simulink model "SWC_FDC_type"  (R2021b)
settings: Solver=FixedStepDiscrete  StartTime=0.0  StopTime=10.0  FixedStep=0.001  RelTol=1e-3
values from neighbouring files (symbols this model uses):
  DID_VCUKey = uint16(0x0202)    [vcu_local_hdr.m]
  DID_XWD = uint16(513)    [vcu_local_hdr.m]
  DIDLen_APSFunConfig = uint16(16)    [vcu_local_hdr.m]
  DIDLen_AutoLock = uint16(1)    [vcu_local_hdr.m]
  DIDLen_DKCKey = uint16(8)    [vcu_local_hdr.m]
  DIDLen_DRLDis = uint16(1)    [vcu_local_hdr.m]
  DIDLen_DynoMode = uint16(1)    [vcu_local_hdr.m]
  DIDLen_FMHTimer = uint16(1)    [vcu_local_hdr.m]
  DIDLen_LFLowPresThre = uint16(1)    [vcu_local_hdr.m]
  DIDLen_LFSensorID = uint16(4)    [vcu_local_hdr.m]
  DIDLen_LRLowPresThre = uint16(1)    [vcu_local_hdr.m]
  DIDLen_LRSensorID = uint16(4)    [vcu_local_hdr.m]
  DIDLen_RFLowPresThre = uint16(1)    [vcu_local_hdr.m]
  DIDLen_RFSensorID = uint16(4)    [vcu_local_hdr.m]
  DIDLen_RRLowPresThre = uint16(1)    [vcu_local_hdr.m]
  DIDLen_RRSensorID = uint16(4)    [vcu_local_hdr.m]
  DIDLen_SensorMode = uint16(1)    [vcu_local_hdr.m]
  DIDLen_TireSize = uint16(16)    [vcu_local_hdr.m]
  DIDLen_TPMSLearnSta = uint16(1)    [vcu_local_hdr.m]
  DIDLen_TurnLampFLThreCurr = uint16(1)    [vcu_local_hdr.m]
  DIDLen_TurnLampFRThreCurr = uint16(1)    [vcu_local_hdr.m]
  DIDLen_TurnLampRLThreCurr = uint16(1)    [vcu_local_hdr.m]
  DIDLen_TurnLampRRThreCurr = uint16(1)    [vcu_local_hdr.m]
  DIDLen_USSConfig = uint16(16)    [vcu_local_hdr.m]
  DIDLen_WhlPres = uint16(4)    [vcu_local_hdr.m]
  DIDLen_WhlSensorBattSta = uint16(1)    [vcu_local_hdr.m]
  DIDLen_WhlTmp = uint16(4)    [vcu_local_hdr.m]
  DIDLen_XWDMode = uint16(1)    [vcu_local_hdr.m]
  DIDNum_APSFunConfig = uint16(0x0903)    [vcu_local_hdr.m]
  DIDNum_AutoLock = uint16(0x0306)    [vcu_local_hdr.m]
  DIDNum_DKCKey = uint16(0x0202)    [vcu_local_hdr.m]
  DIDNum_DRLDis = uint16(0x0307)    [vcu_local_hdr.m]
  DIDNum_DynoMode = uint16(0x0203)    [vcu_local_hdr.m]
  DIDNum_FMHTimer = uint16(0x0305)    [vcu_local_hdr.m]
  DIDNum_LFLowPresThre = uint16(0x0B08)    [vcu_local_hdr.m]
  DIDNum_LFSensorID = uint16(0x0B01)    [vcu_local_hdr.m]
  DIDNum_LRLowPresThre = uint16(0x0B0A)    [vcu_local_hdr.m]
  DIDNum_LRSensorID = uint16(0x0B03)    [vcu_local_hdr.m]
  DIDNum_RFLowPresThre = uint16(0x0B09)    [vcu_local_hdr.m]
  DIDNum_RFSensorID = uint16(0x0B02)    [vcu_local_hdr.m]
  DIDNum_RRLowPresThre = uint16(0x0B0B)    [vcu_local_hdr.m]
  DIDNum_RRSensorID = uint16(0x0B04)    [vcu_local_hdr.m]
  DIDNum_SensorMode = uint16(0x0B0C)    [vcu_local_hdr.m]
  DIDNum_TireSize = uint16(0x0902)    [vcu_local_hdr.m]
  DIDNum_TPMSLearnSta = uint16(0x0B0D)    [vcu_local_hdr.m]
  DIDNum_TurnLampFLThreCurr = uint16(0x0303)    [vcu_local_hdr.m]
  DIDNum_TurnLampFRThreCurr = uint16(0x0301)    [vcu_local_hdr.m]
  DIDNum_TurnLampRLThreCurr = uint16(0x0304)    [vcu_local_hdr.m]
  DIDNum_TurnLampRRThreCurr = uint16(0x0302)    [vcu_local_hdr.m]
  DIDNum_USSConfig = uint16(0x0901)    [vcu_local_hdr.m]
  DIDNum_WhlPres = uint16(0x0B05)    [vcu_local_hdr.m]
  DIDNum_WhlSensorBattSta = uint16(0x0B07)    [vcu_local_hdr.m]
  DIDNum_WhlTmp = uint16(0x0B06)    [vcu_local_hdr.m]
  DIDNum_XWDMode = uint16(0x0201)    [vcu_local_hdr.m]
  DIDVCUKeyLength = uint16(8)    [vcu_local_hdr.m]
  ENUM_DRIVETRAIN_AWD = uint8(  2  )    [vcu_local_hdr.m]
  ENUM_DRIVETRAIN_FWD = uint8(  1  )    [vcu_local_hdr.m]
  ENUM_DRIVETRAIN_RWD = uint8(  0  )    [vcu_local_hdr.m]
  ENUM_TPMSLearnStatus_LEARNED = uint8(  1  )    [vcu_local_hdr.m]
  ENUM_TPMSLearnStatus_LEARNFAIL = uint8(  2  )    [vcu_local_hdr.m]
  ENUM_TPMSLearnStatus_NOTLEARN = uint8(  0  )    [vcu_local_hdr.m]
  ENUM_TPMSSTA_FAT = uint8(  8  )    [vcu_local_hdr.m]
  ENUM_TPMSSTA_LOWBATTERY = uint8(  2  )    [vcu_local_hdr.m]
  FALSE = boolean( 0 )    [vcu_local_hdr.m]
  ONE_INT = uint8(1)    [vcu_local_hdr.m]
  P_boolean = 0.0    [APPTypes.sldd]
  TRUE = boolean( 1 )    [vcu_local_hdr.m]
  ZERO_FLOAT = single(0)    [vcu_local_hdr.m]
  ZERO_INT = uint8(0)    [vcu_local_hdr.m]
undefined symbols (not defined in the file or in its folder): f32_ApsOutVehSpdSig, KHAL_DKCDecryptEnable_flg_ovrdflg, KHAL_DKCDecryptEnable_flg_ovrdval, KHAL_RandomNumberY1_enum, KHAL_RandomNumberY2_enum, KHAL_RandomNumberY_ovrdflg, KHAL_TPMSRESBUTT_flg_ovrdflg, KHAL_TPMSRESBUTT_flg_ovrdval, R_DIDWriteCDD_CSOP_DIDSet_APSFunConfig, R_DIDWriteCDD_CSOP_DIDSet_AutoLock, R_DIDWriteCDD_CSOP_DIDSet_DKCKey, R_DIDWriteCDD_CSOP_DIDSet_DRLDis, R_DIDWriteCDD_CSOP_DIDSet_DynoMode, R_DIDWriteCDD_CSOP_DIDSet_FMHTimer, R_DIDWriteCDD_CSOP_DIDSet_LFLowPresThre, R_DIDWriteCDD_CSOP_DIDSet_LFSensorID, R_DIDWriteCDD_CSOP_DIDSet_LRLowPresThre, R_DIDWriteCDD_CSOP_DIDSet_LRSensorID, R_DIDWriteCDD_CSOP_DIDSet_RFLowPresThre, R_DIDWriteCDD_CSOP_DIDSet_RFSensorID, R_DIDWriteCDD_CSOP_DIDSet_RRLowPresThre, R_DIDWriteCDD_CSOP_DIDSet_RRSensorID, R_DIDWriteCDD_CSOP_DIDSet_SensorMode, R_DIDWriteCDD_CSOP_DIDSet_TireSize, R_DIDWriteCDD_CSOP_DIDSet_TPMSLearnSta, R_DIDWriteCDD_CSOP_DIDSet_TurnLampFLThreCurr, R_DIDWriteCDD_CSOP_DIDSet_TurnLampFRThreCurr, R_DIDWriteCDD_CSOP_DIDSet_TurnLampRLThreCurr, R_DIDWriteCDD_CSOP_DIDSet_TurnLampRRThreCurr, R_DIDWriteCDD_CSOP_DIDSet_USSConfig, R_DIDWriteCDD_CSOP_DIDSet_WhlPres, R_DIDWriteCDD_CSOP_DIDSet_WhlSensorBattSta, R_DIDWriteCDD_CSOP_DIDSet_WhlTmp, R_DIDWriteCDD_CSOP_DIDSet_XWDMode, R_E2E_CAN3_VCU1_CSOP_Write_CAN3_VCU1, R_E2E_CAN3_VCU1_toNIDEC_CSOP_Write_CAN3_VCU1_toNIDEC, R_E2E_CAN4_VCU1_CSOP_Write_CAN4_VCU1, R_FDCCDD_Inner_CSOP_FDC_AppCallSleep, R_HALINCDD_CSOP_PAS_Handler, R_HALINCDD_CSOP_UDS_Main, R_HALOUT_APS_CSOP_ApsOutput, R_HALOUTCDD_CSOP_AppNmStateReq, R_HALOUTCDD_CSOP_SetAcoreRebootCmdACK, R_HALOUTCDD_CSOP_SetSysPwrStat, R_HALOUTCDD_CSOP_SleepRequest, R_IOExpOUT_CDD_CSOP_IOExpSetVal, R_J1939_CAN1_CFGEM1_BAM_CSOP_Write_CAN1_CFGEM1_BAM, R_J1939_CAN1_CFGEM1_DT_CSOP_Write_CAN1_CFGEM1_DT, R_NVMReadCDD_Inner_NVM_ReadOperation, R_NVMWriteCDD_Inner_NVM_WriteOperation, R_UDSCDD_CSOP_DdmRestartOperationCycle, R_WDGCDD_CSOP_Call_Watchdog, R_WDGCDD_CSOP_Call_WDG_AppEnd, R_WDGCDD_CSOP_Call_WDG_AppStart, u16_DIDLen_APSFunConfig, u16_DIDLen_AutoLock, u16_DIDLen_DKCKey, u16_DIDLen_DRLDis, u16_DIDLen_DynoMode, u16_DIDLen_FMHTimer ... (+83)
libraries: simulink x215, FVT_lib x143, hcu_lib x19, hdlsllib x9, app x1, halin x1, halout x1, inp x1, outp x1
(part 11 of 13)

== system SWC_FDC_type/run_SWC_FDC_RxTx_5ms_sys/Halin_CDD/Halin_SYS/Flashfdefog_Verify ==
  In1 : Inport
  Compare To Constant : simulink/Logic and Bit Operations/Compare To Constant  relop=>  const=1  OutDataTypeStr=boolean
  Compare To Constant1 : simulink/Logic and Bit Operations/Compare To Constant  relop=<  const=0  OutDataTypeStr=boolean
  Constant : Constant  Value=ZERO_INT
  Logical Operator : Logic  Operator=OR  AllPortsSameDT=off  OutDataTypeStr=boolean
  Switch : Switch  Criteria=u2 > Threshold
  Out1 : Outport
  wires:
  In1/1 -> Switch/3, Compare To Constant1/1, Compare To Constant/1
  Constant/1 -> Switch/1
  Switch/1 -> Out1/1
  Logical Operator/1 -> Switch/2
  Compare To Constant/1 -> Logical Operator/1
  Compare To Constant1/1 -> Logical Operator/2

== system SWC_FDC_type/run_SWC_FDC_RxTx_5ms_sys/Halin_CDD/Halin_SYS/FlashsigRecircSt_Verify ==
  In1 : Inport
  Compare To Constant : simulink/Logic and Bit Operations/Compare To Constant  relop=>  const=1  OutDataTypeStr=boolean
  Compare To Constant1 : simulink/Logic and Bit Operations/Compare To Constant  relop=<  const=0  OutDataTypeStr=boolean
  Constant : Constant  Value=ZERO_INT
  Logical Operator : Logic  Operator=OR  AllPortsSameDT=off  OutDataTypeStr=boolean
  Switch : Switch  Criteria=u2 > Threshold
  Out1 : Outport
  wires:
  Compare To Constant1/1 -> Logical Operator/2
  Compare To Constant/1 -> Logical Operator/1
  Logical Operator/1 -> Switch/2
  Switch/1 -> Out1/1
  Constant/1 -> Switch/1
  In1/1 -> Compare To Constant/1, Compare To Constant1/1, Switch/3

== system SWC_FDC_type/run_SWC_FDC_RxTx_5ms_sys/Halin_CDD/Halin_SYS/FlashsigSetTempZon1St_Verify ==
  In1 : Inport
  Compare To Constant : simulink/Logic and Bit Operations/Compare To Constant  relop=>  const=32  OutDataTypeStr=boolean
  Compare To Constant1 : simulink/Logic and Bit Operations/Compare To Constant  relop=<  const=17  OutDataTypeStr=boolean
  Constant : Constant  Value=25
  Logical Operator : Logic  Operator=OR  AllPortsSameDT=off  OutDataTypeStr=boolean
  Switch : Switch  Criteria=u2 > Threshold
  Out1 : Outport
  wires:
  In1/1 -> Switch/3, Compare To Constant1/1, Compare To Constant/1
  Constant/1 -> Switch/1
  Switch/1 -> Out1/1
  Logical Operator/1 -> Switch/2
  Compare To Constant/1 -> Logical Operator/1
  Compare To Constant1/1 -> Logical Operator/2

== system SWC_FDC_type/run_SWC_FDC_RxTx_5ms_sys/Halin_CDD/Halin_SYS/FlashsigSetTempZon2StM_Verify ==
  In1 : Inport
  Compare To Constant : simulink/Logic and Bit Operations/Compare To Constant  relop=>  const=32  OutDataTypeStr=boolean
  Compare To Constant1 : simulink/Logic and Bit Operations/Compare To Constant  relop=<  const=17  OutDataTypeStr=boolean
  Constant : Constant  Value=25
  Logical Operator : Logic  Operator=OR  AllPortsSameDT=off  OutDataTypeStr=boolean
  Switch : Switch  Criteria=u2 > Threshold
  Out1 : Outport
  wires:
  Compare To Constant1/1 -> Logical Operator/2
  Compare To Constant/1 -> Logical Operator/1
  Logical Operator/1 -> Switch/2
  Switch/1 -> Out1/1
  Constant/1 -> Switch/1
  In1/1 -> Compare To Constant/1, Compare To Constant1/1, Switch/3

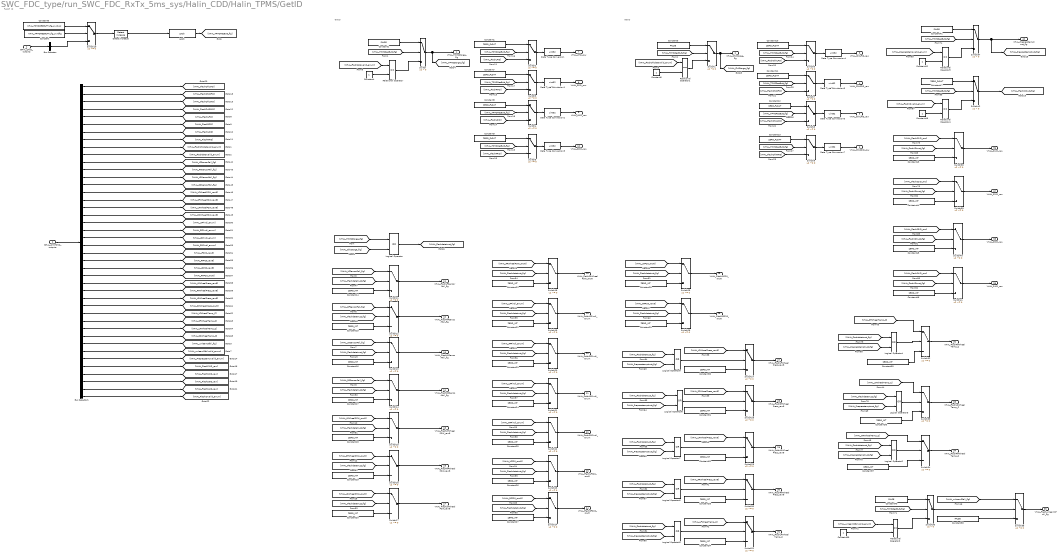
== system SWC_FDC_type/run_SWC_FDC_RxTx_5ms_sys/Halin_CDD/Halin_TPMS/GetID ==
  note: FLASH ID
  note: GetID
  note: GetID
  BHAL_CAN2_outputs : Inport
  BHAL_SYSTPMS_outputs : Inport  Port=2
  Bus Selector : BusSelector  OutputSignals=VHAL_TPMSResButt_flg
  Bus Selector1 : BusSelector  OutputSignals=VHAL_FlashChkLFID_raw,VHAL_FlashChkRFID_raw,VHAL_FlashChkLRID_raw,VHAL_FlashChkRRID_raw,VHAL_FlashLFID_raw,VHAL_FlashRFID_raw,VHAL_FlashLRID_raw,VHAL_FlashRRID_raw,VHAL_Flashchkdatavalid_enum,VHAL_Flashdatavalid_enum,VHAL_LFSensorFail_flg,VHAL_RFSensorFail_flg,VHAL_LRSensorFail_flg,VHAL_RRSensorFail_flg,VHAL_LFWheelPSW_raw8,VHAL_RFWheelPSW_raw8,VHAL_LRWheelPSW_raw8,VHAL_RRWheelPSW_raw8,VHAL_LFPindi_enum,VHAL_RFPindi_enum,VHAL_LRPindi_enum,VHAL_RRPindi_enum,VHAL_LFP20_raw8,VHAL_RFP20_raw8,VHAL_LRP20_raw8,VHAL_RRP20_raw8,VHAL_LFWheelPress_raw8,VHAL_RFWheelPress_raw8,VHAL_LRWheelPress_raw8,VHAL_RRWheelPress_raw8,VHAL_LFWheelTemp_C,VHAL_RFWheelTemp_C,VHAL_LRWheelTemp_C,VHAL_RRWheelTemp_C,VHAL_unlearnSfali_flg,VHAL_unlearnSfailvalid_enum,VHAL_Prepresstempvalid_enum,VHAL_FlashS1ID_raw,VHAL_FlashS2ID_raw,VHAL_FlashS3ID_raw,VHAL_FlashS4ID_raw,VHAL_FlashIDvalid_enum
  Constant : Constant  Value=KHAL_TPMSRESBUTT_flg_ovrdflg
  Constant{1,7..13,47} (9 alike) : Constant  Value=ZERO_FLOAT
  Constant{14..37,43..46} (28 alike) : Constant  Value=ZERO_INT
  Constant{2..3,38,40..41} (5 alike) : Constant  Value=FALSE
  Constant{4..5,39,42,48} (5 alike) : Constant
  Constant6 : Constant  Value=KHAL_TPMSRESBUTT_flg_ovrdval
  Data Type Conversion{,1..7} (8 alike) : DataTypeConversion  OutDataTypeStr=uint32
  Detect Increase : simulink/Logic and Bit Operations/Detect Increase  vinit=0.0  OutDataTypeStr=boolean
  Latch : hcu_lib/Basic_Blocks/Latch
  Logical Operator{,2..9} (9 alike) : Logic  Operator=OR  AllPortsSameDT=off  OutDataTypeStr=boolean
  Relational Operator{,1..4} (5 alike) : RelationalOperator  Operator===  OutDataTypeStr=boolean  RndMeth=Simplest
  Switch{,36..37,42} (4 alike) : Switch  Criteria=u2 > Threshold
  Switch{1..35,38..41} (39 alike) : Switch  Criteria=u2 ~= 0
  VHAL_TPMSStorge_flg : Outport
  VHAL_ChkStorge_flg : Outport  Port=2
  VHAL_ChkLFID_raw : Outport  Port=3
  VHAL_ChkRFID_raw : Outport  Port=4
  VHAL_ChkLRID_raw : Outport  Port=5
  VHAL_ChkRRID_raw : Outport  Port=6
  VHAL_LFID_raw : Outport  Port=7
  VHAL_RFID_raw : Outport  Port=8
  VHAL_LRID_raw : Outport  Port=9
  VHAL_RRID_raw : Outport  Port=10
  VHAL_FlashLFSensorFail_flg : Outport  Port=11
  VHAL_FlashRFSensorFail_flg : Outport  Port=12
  VHAL_FlashLRSensorFail_flg : Outport  Port=13
  VHAL_FlashRRSensorFail_flg : Outport  Port=14
  VHAL_FlashLFWheelPSW_raw8 : Outport  Port=15
  VHAL_FlashRFWheelPSW_raw8 : Outport  Port=16
  VHAL_FlashLRWheelPSW_raw8 : Outport  Port=17
  VHAL_FlashRRWheelPSW_raw8 : Outport  Port=18
  VHAL_FlashLFPindi_enum : Outport  Port=19
  VHAL_FlashRFPindi_enum : Outport  Port=20
  VHAL_FlashLRPindi_enum : Outport  Port=21
  VHAL_FlashRRPindi_enum : Outport  Port=22
  VHAL_FlashLFP20_raw8 : Outport  Port=23
  VHAL_FlashRFP20_raw8 : Outport  Port=24
  VHAL_FlashLRP20_raw8 : Outport  Port=25
  VHAL_FlashRRP20_raw8 : Outport  Port=26
  VHAL_FlashLFWheelPress_raw8 : Outport  Port=27
  VHAL_FlashRFWheelPress_raw8 : Outport  Port=28
  VHAL_FlashLRWheelPress_raw8 : Outport  Port=29
  VHAL_FlashRRWheelPress_raw8 : Outport  Port=30
  VHAL_FlashLFWheelTemp_C : Outport  Port=31
  VHAL_FlashRFWheelTemp_C : Outport  Port=32
  VHAL_FlashLRWheelTemp_C : Outport  Port=33
  VHAL_FlashRRWheelTemp_C : Outport  Port=34
  VHAL_FlashunlearnSfali_flg : Outport  Port=35
  VHAL_S1ID_raw : Outport  Port=36
  VHAL_S2ID_raw : Outport  Port=37
  VHAL_S3ID_raw : Outport  Port=38
  VHAL_S4ID_raw : Outport  Port=39
  VHAL_Prepresstemptrust_flg : Outport  Port=40
  wires:
  BHAL_CAN2_outputs/1 -> Bus Selector/1
  Latch/1 -> [VHAL_TPMSResButt_flg]
  [VHAL_TPMSResButt_flg] -> Switch4/2
  [VHAL_TPMSResButt_flg] -> Switch3/2
  [VHAL_FlashChkLFID] -> Switch6/3
  Switch3/1 -> Data Type Conversion1/1
  [VHAL_FlashRFID] -> Switch3/3
  Constant12/1 -> Switch8/1
  Constant9/1 -> Switch5/1
  [VHAL_FlashRRID] -> Switch5/3
  Constant1/1 -> Switch2/1
  Constant7/1 -> Switch3/1
  [VHAL_TPMSResButt_flg] -> Switch9/2
  [VHAL_TPMSResButt_flg] -> Switch2/2
  [VHAL_FlashLRID] -> Switch4/3
  Constant8/1 -> Switch4/1
  Switch2/1 -> Data Type Conversion/1
  [VHAL_TPMSResButt_flg] -> Switch5/2
  Switch4/1 -> Data Type Conversion2/1
  [VHAL_FlashChkLRID] -> Switch8/3
  [VHAL_FlashChkRRID] -> Switch9/3
  Constant10/1 -> Switch6/1
  Constant11/1 -> Switch7/1
  Switch8/1 -> Data Type Conversion6/1
  [VHAL_TPMSResButt_flg] -> Switch6/2
  Switch6/1 -> Data Type Conversion4/1
  Switch9/1 -> Data Type Conversion7/1
  Constant13/1 -> Switch9/1
  Switch7/1 -> Data Type Conversion5/1
  [VHAL_TPMSResButt_flg] -> Switch8/2
  [VHAL_TPMSResButt_flg] -> Switch7/2
  Switch5/1 -> Data Type Conversion3/1
  [VHAL_FlashChkRFID] -> Switch7/3
  [VHAL_FlashLFID] -> Switch2/3
  Switch10/1 -> Detect Increase/1
  Constant/1 -> Switch10/2
  Constant6/1 -> Switch10/1
  Bus Selector/1 -> Switch10/3  "<VHAL_TPMSResButt_flg>"
  [VHAL_TPMSResButt_flg] -> Switch/2
  Switch/1 -> [VHAL_TPMSStorge_flg], VHAL_TPMSStorge_flg/1
  Constant2/1 -> Switch/1
  Constant3/1 -> Switch1/1
  Switch1/1 -> [VHAL_ChkStorge_flg], VHAL_ChkStorge_flg/1
  [VHAL_TPMSResButt_flg] -> Switch1/2
  [VHAL_Flashdatavalid_enum] -> Relational Operator/1
  Relational Operator/1 -> Switch/3
  Constant4/1 -> Relational Operator/2
  Constant5/1 -> Relational Operator1/2
  Relational Operator1/1 -> Switch1/3
  [VHAL_Flashchkdatavalid_enum] -> Relational Operator1/1
  [VHAL_TPMSStorge_flg] -> Logical Operator/1
  [VHAL_ChkStorge_flg] -> Logical Operator/2
  Logical Operator/1 -> [VHAL_Flashdatatrust_flg]
  [VHAL_Flashdatatrust_flg] -> Switch11/2
  [VHAL_LFSensorFail_flg] -> Switch11/1
  Constant14/1 -> Switch11/3
  Switch11/1 -> VHAL_FlashLFSensorFail_flg/1
  Constant15/1 -> Switch12/3
  [VHAL_Flashdatatrust_flg] -> Switch12/2
  Constant16/1 -> Switch13/3
  [VHAL_Flashdatatrust_flg] -> Switch13/2
  Constant17/1 -> Switch14/3
  [VHAL_Flashdatatrust_flg] -> Switch14/2
  Constant18/1 -> Switch15/3
  [VHAL_Flashdatatrust_flg] -> Switch15/2
  Constant19/1 -> Switch16/3
  [VHAL_Flashdatatrust_flg] -> Switch16/2
  Constant20/1 -> Switch17/3
  [VHAL_Flashdatatrust_flg] -> Switch17/2
  Constant21/1 -> Switch18/3
  [VHAL_Flashdatatrust_flg] -> Switch18/2
  [VHAL_RFSensorFail_flg] -> Switch12/1
  [VHAL_LRSensorFail_flg] -> Switch13/1
  [VHAL_RRSensorFail_flg] -> Switch14/1
  [VHAL_LFWheelPSW_raw8] -> Switch15/1
  [VHAL_RFWheelPSW_raw8] -> Switch16/1
  [VHAL_LRWheelPSW_raw8] -> Switch17/1
  [VHAL_RRWheelPSW_raw8] -> Switch18/1
  Constant22/1 -> Switch19/3
  [VHAL_Flashdatatrust_flg] -> Switch19/2
  Constant23/1 -> Switch20/3
  [VHAL_Flashdatatrust_flg] -> Switch20/2
  Constant24/1 -> Switch21/3
  [VHAL_Flashdatatrust_flg] -> Switch21/2
  Constant25/1 -> Switch22/3
  [VHAL_Flashdatatrust_flg] -> Switch22/2
  [VHAL_LFPindi_enum] -> Switch19/1
  [VHAL_RFPindi_enum] -> Switch20/1
  [VHAL_LRPindi_enum] -> Switch21/1
  [VHAL_RRPindi_enum] -> Switch22/1
  Constant26/1 -> Switch23/3
  [VHAL_Flashdatatrust_flg] -> Switch23/2
  [VHAL_LFP20_raw8] -> Switch23/1
  Constant27/1 -> Switch24/3
  [VHAL_Flashdatatrust_flg] -> Switch24/2
  [VHAL_RFP20_raw8] -> Switch24/1
  Constant28/1 -> Switch25/3
  [VHAL_Flashdatatrust_flg] -> Switch25/2
  [VHAL_LRP20_raw8] -> Switch25/1
  Constant29/1 -> Switch26/3
  [VHAL_Flashdatatrust_flg] -> Switch26/2
  [VHAL_RRP20_raw8] -> Switch26/1
  Constant30/1 -> Switch27/3
  [VHAL_LFWheelPress_raw8] -> Switch27/1
  Constant31/1 -> Switch28/3
  [VHAL_RFWheelPress_raw8] -> Switch28/1
  Constant32/1 -> Switch29/3
  [VHAL_LRWheelPress_raw8] -> Switch29/1
  Constant33/1 -> Switch30/3
  [VHAL_RRWheelPress_raw8] -> Switch30/1
  Constant34/1 -> Switch31/3
  [VHAL_LFWheelTemp_C] -> Switch31/1
  Constant35/1 -> Switch32/3
  [VHAL_RFWheelTemp_C] -> Switch32/1
  Constant36/1 -> Switch33/3
  [VHAL_LRWheelTemp_C] -> Switch33/1
  Constant37/1 -> Switch34/3
  Logical Operator2/1 -> Switch34/2
  Constant38/1 -> Switch35/3
  [VHAL_unlearnSfali_flg] -> Switch35/1
  [VHAL_RRWheelTemp_C] -> Switch34/1
  Switch12/1 -> VHAL_FlashRFSensorFail_flg/1
  Switch13/1 -> VHAL_FlashLRSensorFail_flg/1
  Switch14/1 -> VHAL_FlashRRSensorFail_flg/1
  Switch15/1 -> VHAL_FlashLFWheelPSW_raw8/1
  Switch16/1 -> VHAL_FlashRFWheelPSW_raw8/1
  Switch17/1 -> VHAL_FlashLRWheelPSW_raw8/1
  Switch18/1 -> VHAL_FlashRRWheelPSW_raw8/1
  Switch19/1 -> VHAL_FlashLFPindi_enum/1
  Switch20/1 -> VHAL_FlashRFPindi_enum/1
  Switch21/1 -> VHAL_FlashLRPindi_enum/1
  Switch22/1 -> VHAL_FlashRRPindi_enum/1
  Switch23/1 -> VHAL_FlashLFP20_raw8/1
  Switch24/1 -> VHAL_FlashRFP20_raw8/1
  Switch25/1 -> VHAL_FlashLRP20_raw8/1
  Switch26/1 -> VHAL_FlashRRP20_raw8/1
  Switch27/1 -> VHAL_FlashLFWheelPress_raw8/1
  Switch28/1 -> VHAL_FlashRFWheelPress_raw8/1
  Switch29/1 -> VHAL_FlashLRWheelPress_raw8/1
  Switch30/1 -> VHAL_FlashRRWheelPress_raw8/1
  Switch31/1 -> VHAL_FlashLFWheelTemp_C/1
  Switch32/1 -> VHAL_FlashRFWheelTemp_C/1
  Switch33/1 -> VHAL_FlashLRWheelTemp_C/1
  Switch34/1 -> VHAL_FlashRRWheelTemp_C/1
  [VHAL_unlearnSfailvalid_enum] -> Relational Operator2/1
  Constant39/1 -> Relational Operator2/2
  Constant40/1 -> Switch36/1
  [VHAL_TPMSResButt_flg] -> Switch36/2
  Switch35/1 -> VHAL_FlashunlearnSfali_flg/1
  Switch36/1 -> Switch35/2
  Relational Operator2/1 -> Switch36/3
  Constant42/1 -> Relational Operator3/2
  [VHAL_TPMSResButt_flg] -> Switch37/2
  Constant41/1 -> Switch37/1
  Relational Operator3/1 -> Switch37/3
  [VHAL_Prepresstempvalid_enum] -> Relational Operator3/1
  Switch37/1 -> VHAL_Prepresstemptrust_flg/1, [VHAL_Prepresstemptrust_flg]
  [VHAL_Flashdatatrust_flg] -> Logical Operator2/1
  [VHAL_Prepresstemptrust_flg] -> Logical Operator2/2
  [VHAL_Flashdatatrust_flg] -> Logical Operator3/1
  [VHAL_Prepresstemptrust_flg] -> Logical Operator3/2
  Logical Operator3/1 -> Switch33/2
  [VHAL_Flashdatatrust_flg] -> Logical Operator4/1
  [VHAL_Prepresstemptrust_flg] -> Logical Operator4/2
  Logical Operator4/1 -> Switch32/2
  [VHAL_Flashdatatrust_flg] -> Logical Operator5/1
  [VHAL_Prepresstemptrust_flg] -> Logical Operator5/2
  Logical Operator5/1 -> Switch31/2
  [VHAL_Flashdatatrust_flg] -> Logical Operator6/1
  [VHAL_Prepresstemptrust_flg] -> Logical Operator6/2
  Logical Operator6/1 -> Switch30/2
  [VHAL_Flashdatatrust_flg] -> Logical Operator7/1
  [VHAL_Prepresstemptrust_flg] -> Logical Operator7/2
  Logical Operator7/1 -> Switch29/2
  [VHAL_Flashdatatrust_flg] -> Logical Operator8/1
  [VHAL_Prepresstemptrust_flg] -> Logical Operator8/2
  Logical Operator8/1 -> Switch28/2
  [VHAL_Flashdatatrust_flg] -> Logical Operator9/1
  [VHAL_Prepresstemptrust_flg] -> Logical Operator9/2
  Logical Operator9/1 -> Switch27/2
  Detect Increase/1 -> Latch/1
  Data Type Conversion/1 -> VHAL_LFID_raw/1
  Data Type Conversion1/1 -> VHAL_RFID_raw/1
  Data Type Conversion2/1 -> VHAL_LRID_raw/1
  Data Type Conversion3/1 -> VHAL_RRID_raw/1
  Data Type Conversion4/1 -> VHAL_ChkLFID_raw/1
  Data Type Conversion5/1 -> VHAL_ChkRFID_raw/1
  Data Type Conversion6/1 -> VHAL_ChkLRID_raw/1
  Data Type Conversion7/1 -> VHAL_ChkRRID_raw/1
  Switch42/1 -> [VHAL_FlashIDtrust_flg]
  Constant45/1 -> Switch40/3
  Constant46/1 -> Switch41/3
  Constant44/1 -> Switch39/3
  Switch39/1 -> VHAL_S2ID_raw/1
  [VHAL_FlashS3ID_raw] -> Switch40/1
  [VHAL_FlashS2ID_raw] -> Switch39/1
  [VHAL_FlashS4ID_raw] -> Switch41/1
  Constant43/1 -> Switch38/3
  [VHAL_FlashS1ID_raw] -> Switch38/1
  [VHAL_TPMSResButt_flg] -> Switch42/2
  [VHAL_FlashIDtrust_flg] -> Switch38/2
  Switch41/1 -> VHAL_S4ID_raw/1
  [VHAL_FlashIDtrust_flg] -> Switch39/2
  Constant47/1 -> Switch42/1
  Switch40/1 -> VHAL_S3ID_raw/1
  Constant48/1 -> Relational Operator4/2
  [VHAL_FlashIDtrust_flg] -> Switch41/2
  Switch38/1 -> VHAL_S1ID_raw/1
  [VHAL_FlashIDvalid_enum] -> Relational Operator4/1
  Relational Operator4/1 -> Switch42/3
  [VHAL_FlashIDtrust_flg] -> Switch40/2
  Bus Selector1/35 -> [VHAL_unlearnSfali_flg]  "<VHAL_unlearnSfali_flg>"
  Bus Selector1/4 -> [VHAL_FlashChkRRID]  "<VHAL_FlashChkRRID_raw>"
  Bus Selector1/27 -> [VHAL_LFWheelPress_raw8]  "<VHAL_LFWheelPress_raw8>"
  Bus Selector1/19 -> [VHAL_LFPindi_enum]  "<VHAL_LFPindi_enum>"
  Bus Selector1/21 -> [VHAL_LRPindi_enum]  "<VHAL_LRPindi_enum>"
  Bus Selector1/25 -> [VHAL_LRP20_raw8]  "<VHAL_LRP20_raw8>"
  Bus Selector1/33 -> [VHAL_LRWheelTemp_C]  "<VHAL_LRWheelTemp_C>"
  Bus Selector1/26 -> [VHAL_RRP20_raw8]  "<VHAL_RRP20_raw8>"
  Bus Selector1/18 -> [VHAL_RRWheelPSW_raw8]  "<VHAL_RRWheelPSW_raw8>"
  Bus Selector1/32 -> [VHAL_RFWheelTemp_C]  "<VHAL_RFWheelTemp_C>"
  Bus Selector1/29 -> [VHAL_LRWheelPress_raw8]  "<VHAL_LRWheelPress_raw8>"
  Bus Selector1/8 -> [VHAL_FlashRRID]  "<VHAL_FlashRRID_raw>"
  Bus Selector1/12 -> [VHAL_RFSensorFail_flg]  "<VHAL_RFSensorFail_flg>"
  Bus Selector1/20 -> [VHAL_RFPindi_enum]  "<VHAL_RFPindi_enum>"
  Bus Selector1/11 -> [VHAL_LFSensorFail_flg]  "<VHAL_LFSensorFail_flg>"
  Bus Selector1/24 -> [VHAL_RFP20_raw8]  "<VHAL_RFP20_raw8>"
  Bus Selector1/22 -> [VHAL_RRPindi_enum]  "<VHAL_RRPindi_enum>"
  Bus Selector1/6 -> [VHAL_FlashRFID]  "<VHAL_FlashRFID_raw>"
  Bus Selector1/3 -> [VHAL_FlashChkLRID]  "<VHAL_FlashChkLRID_raw>"
  Bus Selector1/2 -> [VHAL_FlashChkRFID]  "<VHAL_FlashChkRFID_raw>"
  Bus Selector1/37 -> [VHAL_Prepresstempvalid_enum]  "<VHAL_Prepresstempvalid_enum>"
  Bus Selector1/34 -> [VHAL_RRWheelTemp_C]  "<VHAL_RRWheelTemp_C>"
  Bus Selector1/16 -> [VHAL_RFWheelPSW_raw8]  "<VHAL_RFWheelPSW_raw8>"
  Bus Selector1/30 -> [VHAL_RRWheelPress_raw8]  "<VHAL_RRWheelPress_raw8>"
  Bus Selector1/28 -> [VHAL_RFWheelPress_raw8]  "<VHAL_RFWheelPress_raw8>"
  Bus Selector1/14 -> [VHAL_RRSensorFail_flg]  "<VHAL_RRSensorFail_flg>"
  Bus Selector1/38 -> [VHAL_FlashS1ID_raw]  "<VHAL_FlashS1ID_raw>"
  Bus Selector1/41 -> [VHAL_FlashS4ID_raw]  "<VHAL_FlashS4ID_raw>"
  Bus Selector1/10 -> [VHAL_Flashdatavalid_enum]  "<VHAL_Flashdatavalid_enum>"
  Bus Selector1/15 -> [VHAL_LFWheelPSW_raw8]  "<VHAL_LFWheelPSW_raw8>"
  Bus Selector1/5 -> [VHAL_FlashLFID]  "<VHAL_FlashLFID_raw>"
  Bus Selector1/39 -> [VHAL_FlashS2ID_raw]  "<VHAL_FlashS2ID_raw>"
  BHAL_SYSTPMS_outputs/1 -> Bus Selector1/1
  Bus Selector1/9 -> [VHAL_Flashchkdatavalid_enum]  "<VHAL_Flashchkdatavalid_enum>"
  Bus Selector1/1 -> [VHAL_FlashChkLFID]  "<VHAL_FlashChkLFID_raw>"
  Bus Selector1/7 -> [VHAL_FlashLRID]  "<VHAL_FlashLRID_raw>"
  Bus Selector1/36 -> [VHAL_unlearnSfailvalid_enum]  "<VHAL_unlearnSfailvalid_enum>"
  Bus Selector1/23 -> [VHAL_LFP20_raw8]  "<VHAL_LFP20_raw8>"
  Bus Selector1/40 -> [VHAL_FlashS3ID_raw]  "<VHAL_FlashS3ID_raw>"
  Bus Selector1/13 -> [VHAL_LRSensorFail_flg]  "<VHAL_LRSensorFail_flg>"
  Bus Selector1/42 -> [VHAL_FlashIDvalid_enum]  "<VHAL_FlashIDvalid_enum>"
  Bus Selector1/31 -> [VHAL_LFWheelTemp_C]  "<VHAL_LFWheelTemp_C>"
  Bus Selector1/17 -> [VHAL_LRWheelPSW_raw8]  "<VHAL_LRWheelPSW_raw8>"

== system SWC_FDC_type/run_SWC_FDC_RxTx_5ms_sys/Halin_CDD/Halin_TPMS/Subsystem ==
  note: Custom State Judgement
  note: Data Output
  note: Data Valid Judge
  TPMS_DataIn_flg : Inport
  TPMS_RawData : Inport  Port=2
  Add : Sum  Inputs=++++
  Bit Shift : hdlsllib/Logic and Bit Operations/Bit Shift  mode=Shift Left Logical  N=24
  Bit Shift1 : hdlsllib/Logic and Bit Operations/Bit Shift  mode=Shift Left Logical  N=16
  Bit Shift3 : hdlsllib/Logic and Bit Operations/Bit Shift  mode=Shift Left Logical  N=8
  Bitwise NOT : simulink/Logic and Bit Operations/Bitwise Operator  logicop=NOT  UseBitMask=off  BitMask=bin2dec('11011001')  BitMaskRealWorld=Stored Integer
  CRC8_Caculation : Subsystem
  Constant2 : Constant  Value=ENUM_TPMSSTA_LOWBATTERY
  Constant3 : Constant  Value=ENUM_TPMSSTA_FAT
  Constant4 : Constant  Value=TRUE
  Constant5 : Constant  Value=FALSE
  Constant6 : Constant  Value=FALSE
  Constant7 : Constant  Value=TRUE
  Constant8 : Constant  Value=FALSE
  Constant9 : Constant  Value=TRUE
  Data Type Conversion : DataTypeConversion  OutDataTypeStr=uint32
  Data Type Conversion1 : DataTypeConversion  OutDataTypeStr=uint8
  Data Type Conversion2 : DataTypeConversion  OutDataTypeStr=uint8
  Data Type Conversion3 : DataTypeConversion  OutDataTypeStr=uint32
  Data Type Conversion4 : DataTypeConversion  OutDataTypeStr=uint32
  Demux : Demux  Outputs=9
  Demux1 : Demux  Outputs=10
  Equal{,1..3} (4 alike) : RelationalOperator  Operator===  OutDataTypeStr=boolean  RndMeth=Simplest
  Logical Operator : Logic  Inputs=3  AllPortsSameDT=off  OutDataTypeStr=boolean
  Mux : Mux  Inputs=10
  Mux1 : Mux  Inputs=8
  Switch{,1..3} (4 alike) : Switch  Criteria=u2 ~= 0
  Unit Delay : UnitDelay  SampleTime=-1  HasFrameUpgradeWarning=on
  VHAL_TPMSDataIn_flg : Outport
  VHAL_TPMSID_raw : Outport  Port=2
  VHAL_TPMSPressure_raw : Outport  Port=3
  VHAL_TPMSTemp_raw : Outport  Port=4
  VHAL_TPMSSta_enum : Outport  Port=5
  VHAL_TPMSPressureMi_raw : Outport  Port=6
  VHAL_TPMSCRC_crc : Outport  Port=7
  VHAL_TPMSCRCCalc_crc : Outport  Port=8
  VHAL_TPMSFAT_flg : Outport  Port=9
  VHAL_TPMSBattLow_flg : Outport  Port=10
  wires:
  TPMS_DataIn_flg/1 -> Data Type Conversion2/1
  [TPMSData] -> Demux/1
  Bit Shift/1 -> Add/1
  Bit Shift1/1 -> Add/2
  Bit Shift3/1 -> Add/3
  Add/1 -> VHAL_TPMSID_raw/1
  Demux/5 -> [Pressure]  "Pressure"
  Demux/7 -> [Status]  "Sta"
  Demux/8 -> [PressureMirror]  "PressureMirror"
  Demux/9 -> [CRC]  "CRC"
  Demux/1 -> [ID4]  "ID4"
  Demux/2 -> [ID3]  "ID3"
  Demux/3 -> [ID2]  "ID2"
  Demux/4 -> [ID1]  "ID1"
  Demux/6 -> [Temp]  "Temp"
  [Pressure] -> Bitwise NOT/1
  Bitwise NOT/1 -> Equal/1
  [PressureMirror] -> Equal/2
  [ID4] -> Mux1/1
  [ID3] -> Mux1/2
  [ID2] -> Mux1/3
  [ID1] -> Mux1/4
  [Pressure] -> Mux1/5
  [Temp] -> Mux1/6
  [Status] -> Mux1/7
  [PressureMirror] -> Mux1/8
  Mux1/1 -> CRC8_Caculation/1(MsgData)
  [CRC] -> Equal1/2
  Equal1/1 -> Logical Operator/1
  Equal/1 -> Logical Operator/2
  Logical Operator/1 -> [DataValid_flg]
  [DataValid_flg] -> Switch/2
  Mux/1 -> Switch/1
  Switch/1 -> Unit Delay/1, Demux1/1
  Unit Delay/1 -> Switch/3
  Data Type Conversion1/1 -> [TPMSData]
  Data Type Conversion2/1 -> [Data_in]
  CRC8_Caculation/1(CRCout) -> [CRC_Calc], Equal1/1  "CRC_Calc"
  Switch1/1 -> VHAL_TPMSFAT_flg/1
  [VHAL_TPMSSta_enum] -> Equal2/1
  Constant3/1 -> Equal2/2
  Equal2/1 -> Switch1/2
  Constant4/1 -> Switch1/1
  Constant5/1 -> Switch1/3
  Constant8/1 -> Switch2/3
  [VHAL_TPMSSta_enum] -> Equal3/1
  Constant7/1 -> Switch2/1
  Switch2/1 -> VHAL_TPMSBattLow_flg/1
  Equal3/1 -> Switch2/2
  Constant2/1 -> Equal3/2
  [Data_in] -> Logical Operator/3
  [DataValid_flg] -> Switch3/2
  Switch3/1 -> VHAL_TPMSDataIn_flg/1
  Constant6/1 -> Switch3/3
  Constant9/1 -> Switch3/1
  [ID4] -> Mux/1
  [ID3] -> Mux/2
  [ID2] -> Mux/3
  [ID1] -> Mux/4
  [Pressure] -> Mux/5
  [Temp] -> Mux/6
  [Status] -> Mux/7
  [PressureMirror] -> Mux/8
  [CRC] -> Mux/9
  [CRC_Calc] -> Mux/10
  Demux1/10 -> VHAL_TPMSCRCCalc_crc/1
  Demux1/9 -> VHAL_TPMSCRC_crc/1
  Demux1/8 -> VHAL_TPMSPressureMi_raw/1
  Demux1/7 -> [VHAL_TPMSSta_enum], VHAL_TPMSSta_enum/1
  Demux1/6 -> VHAL_TPMSTemp_raw/1
  Demux1/5 -> VHAL_TPMSPressure_raw/1
  Demux1/1 -> Data Type Conversion/1
  Demux1/2 -> Data Type Conversion3/1
  Demux1/3 -> Data Type Conversion4/1
  Data Type Conversion/1 -> Bit Shift/1
  Data Type Conversion3/1 -> Bit Shift1/1
  Data Type Conversion4/1 -> Bit Shift3/1
  Demux1/4 -> Add/4
  TPMS_RawData/1 -> Data Type Conversion1/1

== system SWC_FDC_type/run_SWC_FDC_RxTx_5ms_sys/OUTP_AFTER/DID_list/uint32Touint8Array ==
  In1 : Inport
  Bitwise AND1 : simulink/Logic and Bit Operations/Bitwise Operator  logicop=AND  UseBitMask=on  BitMask=bin2dec('00000000000000000000000011111111')  BitMaskRealWorld=Stored Integer
  Bitwise AND2 : simulink/Logic and Bit Operations/Bitwise Operator  logicop=AND  UseBitMask=on  BitMask=bin2dec('00000000000000001111111100000000')  BitMaskRealWorld=Stored Integer
  Bitwise AND3 : simulink/Logic and Bit Operations/Bitwise Operator  logicop=AND  UseBitMask=on  BitMask=bin2dec('00000000111111110000000000000000')  BitMaskRealWorld=Stored Integer
  Bitwise AND4 : simulink/Logic and Bit Operations/Bitwise Operator  logicop=AND  UseBitMask=on  BitMask=bin2dec('11111111000000000000000000000000')  BitMaskRealWorld=Stored Integer
  Data Type Conversion{1,3..5} (4 alike) : DataTypeConversion  OutDataTypeStr=uint8
  Data Type Conversion2 : DataTypeConversion  OutDataTypeStr=uint32
  Mux2 : Mux
  Shift Arithmetic39 : ArithShift  BitShiftNumber=8  BitShiftDirection=Right
  Shift Arithmetic40 : ArithShift  BitShiftNumber=16  BitShiftDirection=Right
  Shift Arithmetic41 : ArithShift  BitShiftNumber=24  BitShiftDirection=Right
  Out1 : Outport
  wires:
  Bitwise AND4/1 -> Shift Arithmetic41/1
  Bitwise AND1/1 -> Data Type Conversion1/1
  Shift Arithmetic40/1 -> Data Type Conversion4/1
  Shift Arithmetic41/1 -> Data Type Conversion3/1
  Mux2/1 -> Out1/1
  In1/1 -> Data Type Conversion2/1
  Bitwise AND3/1 -> Shift Arithmetic40/1
  Shift Arithmetic39/1 -> Data Type Conversion5/1
  Data Type Conversion3/1 -> Mux2/1
  Bitwise AND2/1 -> Shift Arithmetic39/1
  Data Type Conversion2/1 -> Bitwise AND4/1, Bitwise AND3/1, Bitwise AND1/1, Bitwise AND2/1
  Data Type Conversion5/1 -> Mux2/3
  Data Type Conversion4/1 -> Mux2/2
  Data Type Conversion1/1 -> Mux2/4

== system SWC_FDC_type/run_SWC_FDC_RxTx_5ms_sys/OUTP_AFTER/DID_list/uint32Touint8Array1 ==
  In1 : Inport
  Bitwise AND1 : simulink/Logic and Bit Operations/Bitwise Operator  logicop=AND  UseBitMask=on  BitMask=bin2dec('00000000000000000000000011111111')  BitMaskRealWorld=Stored Integer
  Bitwise AND2 : simulink/Logic and Bit Operations/Bitwise Operator  logicop=AND  UseBitMask=on  BitMask=bin2dec('00000000000000001111111100000000')  BitMaskRealWorld=Stored Integer
  Bitwise AND3 : simulink/Logic and Bit Operations/Bitwise Operator  logicop=AND  UseBitMask=on  BitMask=bin2dec('00000000111111110000000000000000')  BitMaskRealWorld=Stored Integer
  Bitwise AND4 : simulink/Logic and Bit Operations/Bitwise Operator  logicop=AND  UseBitMask=on  BitMask=bin2dec('11111111000000000000000000000000')  BitMaskRealWorld=Stored Integer
  Data Type Conversion{1,3..5} (4 alike) : DataTypeConversion  OutDataTypeStr=uint8
  Data Type Conversion2 : DataTypeConversion  OutDataTypeStr=uint32
  Mux2 : Mux
  Shift Arithmetic39 : ArithShift  BitShiftNumber=8  BitShiftDirection=Right
  Shift Arithmetic40 : ArithShift  BitShiftNumber=16  BitShiftDirection=Right
  Shift Arithmetic41 : ArithShift  BitShiftNumber=24  BitShiftDirection=Right
  Out1 : Outport
  wires:
  Data Type Conversion1/1 -> Mux2/4
  Data Type Conversion4/1 -> Mux2/2
  Data Type Conversion5/1 -> Mux2/3
  Data Type Conversion2/1 -> Bitwise AND2/1, Bitwise AND1/1, Bitwise AND3/1, Bitwise AND4/1
  Bitwise AND2/1 -> Shift Arithmetic39/1
  Data Type Conversion3/1 -> Mux2/1
  Shift Arithmetic39/1 -> Data Type Conversion5/1
  Bitwise AND3/1 -> Shift Arithmetic40/1
  In1/1 -> Data Type Conversion2/1
  Mux2/1 -> Out1/1
  Shift Arithmetic41/1 -> Data Type Conversion3/1
  Shift Arithmetic40/1 -> Data Type Conversion4/1
  Bitwise AND1/1 -> Data Type Conversion1/1
  Bitwise AND4/1 -> Shift Arithmetic41/1

== system SWC_FDC_type/run_SWC_FDC_RxTx_5ms_sys/OUTP_AFTER/DID_list/uint32Touint8Array2 ==
  In1 : Inport
  Bitwise AND1 : simulink/Logic and Bit Operations/Bitwise Operator  logicop=AND  UseBitMask=on  BitMask=bin2dec('00000000000000000000000011111111')  BitMaskRealWorld=Stored Integer
  Bitwise AND2 : simulink/Logic and Bit Operations/Bitwise Operator  logicop=AND  UseBitMask=on  BitMask=bin2dec('00000000000000001111111100000000')  BitMaskRealWorld=Stored Integer
  Bitwise AND3 : simulink/Logic and Bit Operations/Bitwise Operator  logicop=AND  UseBitMask=on  BitMask=bin2dec('00000000111111110000000000000000')  BitMaskRealWorld=Stored Integer
  Bitwise AND4 : simulink/Logic and Bit Operations/Bitwise Operator  logicop=AND  UseBitMask=on  BitMask=bin2dec('11111111000000000000000000000000')  BitMaskRealWorld=Stored Integer
  Data Type Conversion{1,3..5} (4 alike) : DataTypeConversion  OutDataTypeStr=uint8
  Data Type Conversion2 : DataTypeConversion  OutDataTypeStr=uint32
  Mux2 : Mux
  Shift Arithmetic39 : ArithShift  BitShiftNumber=8  BitShiftDirection=Right
  Shift Arithmetic40 : ArithShift  BitShiftNumber=16  BitShiftDirection=Right
  Shift Arithmetic41 : ArithShift  BitShiftNumber=24  BitShiftDirection=Right
  Out1 : Outport
  wires:
  Bitwise AND4/1 -> Shift Arithmetic41/1
  Bitwise AND1/1 -> Data Type Conversion1/1
  Shift Arithmetic40/1 -> Data Type Conversion4/1
  Shift Arithmetic41/1 -> Data Type Conversion3/1
  Mux2/1 -> Out1/1
  In1/1 -> Data Type Conversion2/1
  Bitwise AND3/1 -> Shift Arithmetic40/1
  Shift Arithmetic39/1 -> Data Type Conversion5/1
  Data Type Conversion3/1 -> Mux2/1
  Bitwise AND2/1 -> Shift Arithmetic39/1
  Data Type Conversion2/1 -> Bitwise AND4/1, Bitwise AND3/1, Bitwise AND1/1, Bitwise AND2/1
  Data Type Conversion5/1 -> Mux2/3
  Data Type Conversion4/1 -> Mux2/2
  Data Type Conversion1/1 -> Mux2/4

== system SWC_FDC_type/run_SWC_FDC_RxTx_5ms_sys/OUTP_AFTER/DID_list/uint32Touint8Array3 ==
  In1 : Inport
  Bitwise AND1 : simulink/Logic and Bit Operations/Bitwise Operator  logicop=AND  UseBitMask=on  BitMask=bin2dec('00000000000000000000000011111111')  BitMaskRealWorld=Stored Integer
  Bitwise AND2 : simulink/Logic and Bit Operations/Bitwise Operator  logicop=AND  UseBitMask=on  BitMask=bin2dec('00000000000000001111111100000000')  BitMaskRealWorld=Stored Integer
  Bitwise AND3 : simulink/Logic and Bit Operations/Bitwise Operator  logicop=AND  UseBitMask=on  BitMask=bin2dec('00000000111111110000000000000000')  BitMaskRealWorld=Stored Integer
  Bitwise AND4 : simulink/Logic and Bit Operations/Bitwise Operator  logicop=AND  UseBitMask=on  BitMask=bin2dec('11111111000000000000000000000000')  BitMaskRealWorld=Stored Integer
  Data Type Conversion{1,3..5} (4 alike) : DataTypeConversion  OutDataTypeStr=uint8
  Data Type Conversion2 : DataTypeConversion  OutDataTypeStr=uint32
  Mux2 : Mux
  Shift Arithmetic39 : ArithShift  BitShiftNumber=8  BitShiftDirection=Right
  Shift Arithmetic40 : ArithShift  BitShiftNumber=16  BitShiftDirection=Right
  Shift Arithmetic41 : ArithShift  BitShiftNumber=24  BitShiftDirection=Right
  Out1 : Outport
  wires:
  Data Type Conversion1/1 -> Mux2/4
  Data Type Conversion4/1 -> Mux2/2
  Data Type Conversion5/1 -> Mux2/3
  Data Type Conversion2/1 -> Bitwise AND2/1, Bitwise AND1/1, Bitwise AND3/1, Bitwise AND4/1
  Bitwise AND2/1 -> Shift Arithmetic39/1
  Data Type Conversion3/1 -> Mux2/1
  Shift Arithmetic39/1 -> Data Type Conversion5/1
  Bitwise AND3/1 -> Shift Arithmetic40/1
  In1/1 -> Data Type Conversion2/1
  Mux2/1 -> Out1/1
  Shift Arithmetic41/1 -> Data Type Conversion3/1
  Shift Arithmetic40/1 -> Data Type Conversion4/1
  Bitwise AND1/1 -> Data Type Conversion1/1
  Bitwise AND4/1 -> Shift Arithmetic41/1
